simulink model "final"  (R2023a)
settings: Solver=VariableStepAuto  StartTime=0.0  StopTime=1.5  RelTol=1e-3
libraries: dspfdesign x6, spspowerguiLib x1
settings Model: SimulationMode=accelerator  Creator=04  LastModifiedBy=23688
settings SolverCC: AlgebraicLoopSolver=TrustRegion
settings DataIOCC: ReturnWorkspaceOutputs=off
settings DebuggingCC: UnconnectedInputMsg=warning  UnconnectedOutputMsg=warning  UnconnectedLineMsg=warning
settings ModelReferenceCC: EnableRefExpFcnMdlSchedulingChecks=on
settings RTWCC: DLArmComputeVersion=19.05

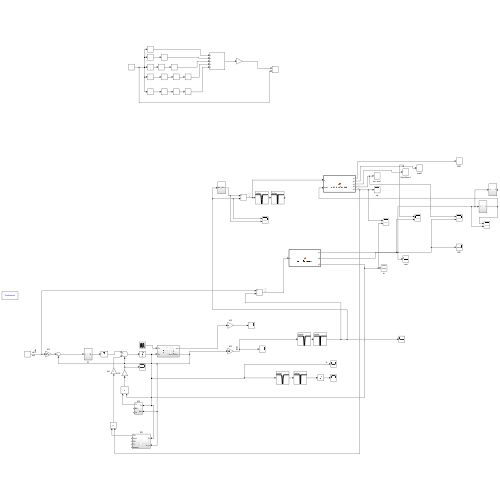
[thumbnail: Simulink's stored preview of the top-level diagram]
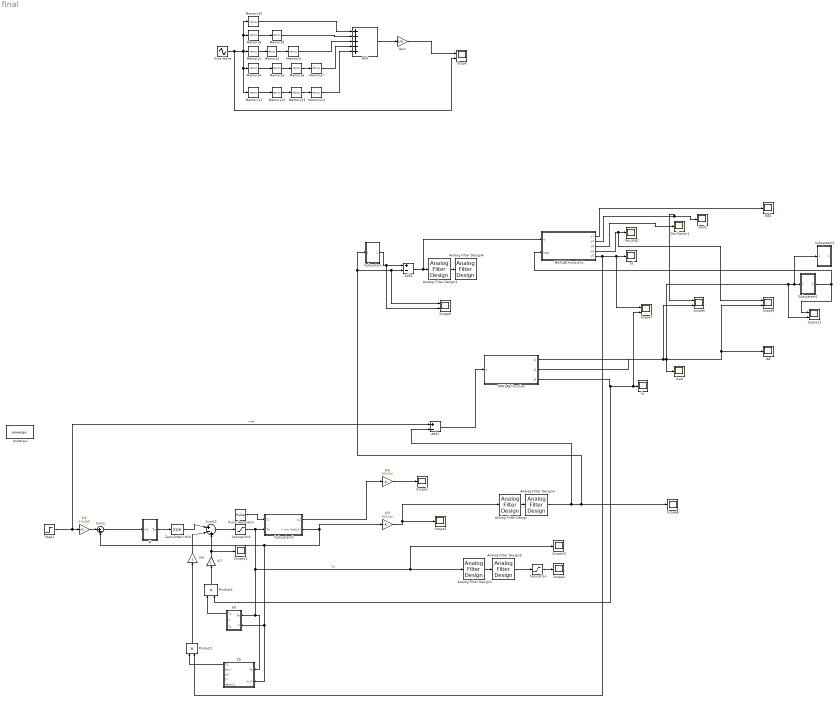
== system final ==
  Add : Sum  Inputs=+++++
  Add1 : Sum  Inputs=+-
  Add2 : Sum  Inputs=+-
  Analog Filter Design : dspfdesign/Analog Filter Design  method=Butterworth  filttype=Bandstop  N=12  Wlo=700*2*pi  Whi=1300*2*pi  Rp=2  Rs=40
  Analog Filter Design1 : dspfdesign/Analog Filter Design  method=Butterworth  filttype=Bandstop  N=2  Wlo=700*2*pi  Whi=1300*2*pi  Rp=2  Rs=40
  Analog Filter Design2 : dspfdesign/Analog Filter Design  method=Butterworth  filttype=Bandstop  N=12  Wlo=700*2*pi  Whi=1300*2*pi  Rp=2  Rs=40
  Analog Filter Design3 : dspfdesign/Analog Filter Design  method=Butterworth  filttype=Bandstop  N=12  Wlo=900*2*pi  Whi=1100*2*pi  Rp=2  Rs=40
  Analog Filter Design4 : dspfdesign/Analog Filter Design  method=Butterworth  filttype=Bandstop  N=12  Wlo=900*2*pi  Whi=1100*2*pi  Rp=2  Rs=40
  Analog Filter Design5 : dspfdesign/Analog Filter Design  method=Butterworth  filttype=Bandstop  N=2  Wlo=950*2*pi  Whi=1050*2*pi  Rp=2  Rs=40
  Gain : Gain  Gain=1/5
  IAE : Scope
  IAE1 : Scope
  Iae_avg1 : Scope
  KR : Subsystem
  Ki2 : Gain  Gain=2*pi/60
  Ki3 : Gain  Gain=60/2/pi
  Ki5 : Gain  Gain=60/2/pi
  Ki6 : Gain
  Ki7 : Gain
  MATLAB Function : MATLAB Function  TreatAsAtomicUnit=on
  MATLAB Function1 : MATLAB Function  TreatAsAtomicUnit=on
  Memory{1..14} (14 alike) : Memory  InitialCondition=0.001
  Oscillation1 : Scope
  PI : Subsystem
  Product1 : Product
  Product2 : Product
  Pulse Generator : DiscretePulseGenerator  PulseType=Time based  Amplitude=2.39*0.5*1  Period=0.8  PulseWidth=50  PhaseDelay=0.4
  Saturation : Saturate  UpperLimit=2.39*3  LowerLimit=-2.39*3  ZeroCross=off
  Saturation3 : Saturate  UpperLimit=2.39*3  LowerLimit=-2.39*3
  Scope{,5..7,9,11} (6 alike) : Scope  NumInputPorts=2
  Scope{1..3,8,10,12} (6 alike) : Scope
  Sine Wave : Sin  Frequency=1000*2*pi  SampleTime=0
  Step2 : Step  Time=0.01  After=1000  SampleTime=0
  Subsystem : Subsystem
  Subsystem1 : Subsystem
  Subsystem2 : Subsystem
  Subsystem3 : Subsystem
  Sum13 : Sum  Inputs=|+-+
  Sum2 : Sum  Inputs=|+-
  ZD : Subsystem
  Zero-Order Hold : ZeroOrderHold  SampleTime=0.0005
  kr : Scope
  load : Scope
  load1 : Scope
  powergui : spspowerguiLib/powergui  Priority=1  SimulationMode=Continuous  SampleTime=50e-6  frequency=60  Iterations=50  frequencyindice=60  Pbase=100e6  ErrMax=1e-4  UnitsV=kV  UnitsW=MW  buscounter=0  FunctionMessages=off  echomessages=off  EnableUseOfTLC=off  CurrentSourceSwitches=off  DisableSnubberDevices=off  DisableRonSwitches=off  DisableVfSwitches=off  DisplayEquations=off  AutomaticDiscreteSolvers=off  SolverType=Tustin/Backward Euler (TBE)  Interpol=off  ExternalGateDelay=off  methode=off  Ts=100  x0status=blocks  SPID=on  SwTol=0  HookPort=off  NonlinearTolerance=1e-4  nMaxIteration=100  ContinueOnMaxIteration=off  RestoreLinks=warning  ResistiveCurrentMeasurement=off  Frange=[0:2:500]  Ylog=off  Xlog=on  ShowGrid=off  save=off  variable=ZData  structure=0  ZoomFFT=off  StartTime=0.0  cycles=1  DisplayStyle=1  fundamental=60  FreqAxis=off  MaxFrequency=1000  frequencyindicesteady=1  RmsSteady=1  display=off
  zd : Scope
  wires:
  Memory1/1 -> Memory2/1
  Memory2/1 -> Memory3/1
  Memory4/1 -> Memory5/1
  Memory5/1 -> Memory6/1
  Memory6/1 -> Memory7/1
  Memory8/1 -> Memory9/1
  Memory10/1 -> Add/1
  Memory9/1 -> Add/2
  Memory3/1 -> Add/3
  Memory7/1 -> Add/4
  Memory14/1 -> Add/5
  Memory13/1 -> Memory14/1
  Memory12/1 -> Memory13/1
  Memory11/1 -> Memory12/1
  Sine Wave/1 -> Scope/2, Memory10/1, Memory8/1, Memory11/1, Memory4/1, Memory1/1
  Add/1 -> Gain/1
  Gain/1 -> Scope/1
  Ki5/1 -> Scope1/1
  Step2/1 -> Add1/1, Ki2/1  "wref"
  Add1/1 -> MATLAB Function/1(e)
  Saturation3/1 -> Subsystem2/2(Te), Scope10/1, Analog Filter Design1/1, ZD/1(Te), KR/1(Te)  "Te"
  MATLAB Function/1(y1) -> IAE/1, Scope6/2
  Analog Filter Design/1 -> Analog Filter Design3/1
  Sum13/1 -> Saturation3/1
  Ki7/1 -> Sum13/3, Scope12/1
  Product1/1 -> Ki6/1
  Ki6/1 -> Sum13/2
  Product2/1 -> Ki7/1
  Ki3/1 -> Analog Filter Design/1, Scope3/1
  Ki2/1 -> Sum2/1
  MATLAB Function1/2(y2) -> Scope5/1, load1/1
  MATLAB Function1/3(y3) -> Oscillation1/1
  MATLAB Function1/4(y4) -> Scope6/1, Iae_avg1/1
  MATLAB Function1/1(y1) -> IAE1/1
  MATLAB Function1/5(y5) -> Scope7/1, zd/1, Product1/2
  Analog Filter Design2/1 -> Analog Filter Design4/1
  Add2/1 -> MATLAB Function1/1(e), Analog Filter Design2/1
  MATLAB Function/3(y3) -> Scope7/2, kr/1, Product2/2
  Subsystem/1(wm_filter) -> Scope9/2, Add2/1
  Analog Filter Design3/1 -> Scope8/1, Scope9/1, Add2/2, Subsystem/1(In1), Add1/2
  MATLAB Function/2(y2) -> Scope5/2, load/1, Scope11/2, Subsystem3/1(In1), Subsystem1/1(In1)
  Subsystem1/1(Out1) -> Scope11/1, MATLAB Function1/2(load)
  Analog Filter Design1/1 -> Analog Filter Design5/1
  Analog Filter Design5/1 -> Saturation/1
  Saturation/1 -> Scope2/1
  Sum2/1 -> PI/1(In1)
  Subsystem2/2(< wm (rad/s)>) -> Ki3/1, Sum2/2, ZD/2(w_m), KR/2(Wm)
  Pulse Generator/1 -> Subsystem2/1(TL)
  Subsystem2/1(w2) -> Ki5/1
  KR/1(TL) -> Product2/1
  ZD/1(TS) -> Product1/1
  PI/1(Te) -> Zero-Order Hold/1
  Zero-Order Hold/1 -> Sum13/1

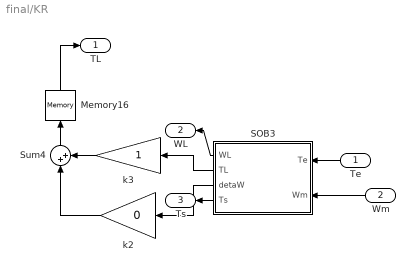
== system final/KR ==
  Te : Inport
  Wm : Inport  Port=2
  Memory16 : Memory
  SOB3 : Subsystem
  Sum4 : Sum  Inputs=|++
  k2 : Gain  Gain=0
  k3 : Gain
  TL : Outport
  WL : Outport  Port=2
  Ts : Outport  Port=3
  wires:
  Sum4/1 -> Memory16/1
  Memory16/1 -> TL/1
  SOB3/3(detaW) -> k2/1
  SOB3/1(WL) -> WL/1
  SOB3/4(Ts) -> Ts/1
  SOB3/2(TL) -> k3/1
  k3/1 -> Sum4/2
  k2/1 -> Sum4/1
  Wm/1 -> SOB3/2(Wm)
  Te/1 -> SOB3/1(Te)

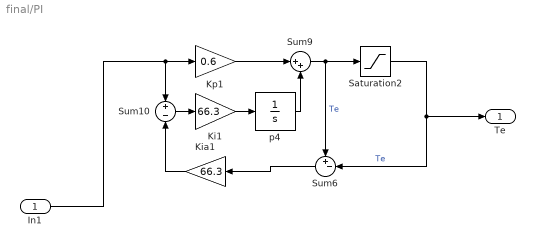
== system final/PI ==
  In1 : Inport
  Ki1 : Gain  Gain=66.3
  Kia1 : Gain  Gain=66.3
  Kp1 : Gain  Gain=0.6
  Saturation2 : Saturate  UpperLimit=2.39*3  LowerLimit=-2.39*3
  Sum10 : Sum  Inputs=+|-
  Sum6 : Sum  Inputs=+-|
  Sum9 : Sum  Inputs=|++
  p4 : TransferFcn  Denominator=[1 0]
  Te : Outport
  wires:
  Kia1/1 -> Sum10/2
  Sum6/1 -> Kia1/1
  Sum10/1 -> Ki1/1
  Kp1/1 -> Sum9/1
  Saturation2/1 -> Te/1, Sum6/2  "Te"
  Sum9/1 -> Sum6/1, Saturation2/1  "Te"
  p4/1 -> Sum9/2
  Ki1/1 -> p4/1
  In1/1 -> Kp1/1, Sum10/1

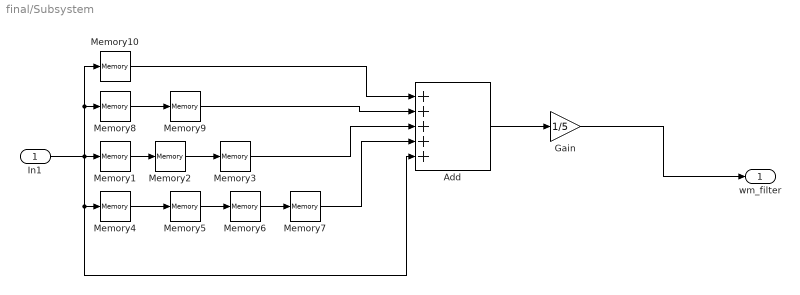
== system final/Subsystem ==
  In1 : Inport
  Add : Sum  Inputs=+++++
  Gain : Gain  Gain=1/5
  Memory{1..10} (10 alike) : Memory
  wm_filter : Outport
  wires:
  In1/1 -> Memory10/1, Memory8/1, Add/5, Memory4/1, Memory1/1
  Memory1/1 -> Memory2/1
  Memory4/1 -> Memory5/1
  Add/1 -> Gain/1
  Memory8/1 -> Memory9/1
  Memory5/1 -> Memory6/1
  Memory9/1 -> Add/2
  Memory7/1 -> Add/4
  Memory6/1 -> Memory7/1
  Memory10/1 -> Add/1
  Memory3/1 -> Add/3
  Memory2/1 -> Memory3/1
  Gain/1 -> wm_filter/1

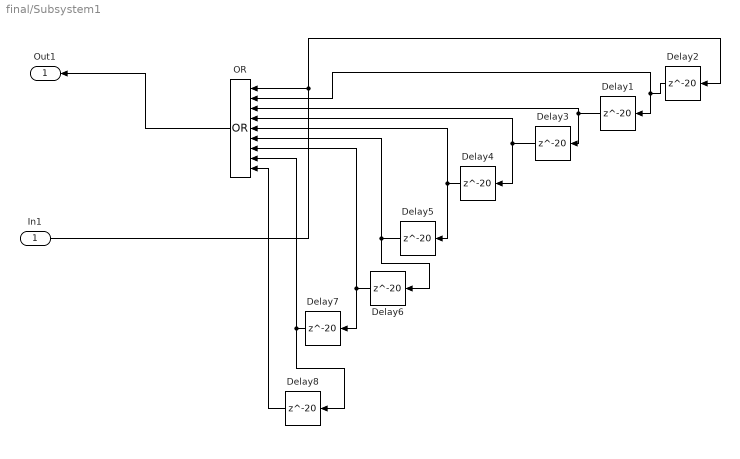
== system final/Subsystem1 ==
  In1 : Inport
  Delay{1..8} (8 alike) : Delay  DelayLength=20
  OR : Logic  Operator=OR  Inputs=9  IconShape=distinctive  AllPortsSameDT=off  OutDataTypeStr=boolean
  Out1 : Outport
  wires:
  Delay2/1 -> Delay1/1, OR/2
  Delay4/1 -> Delay5/1, OR/5
  Delay3/1 -> Delay4/1, OR/4
  Delay1/1 -> OR/3, Delay3/1
  In1/1 -> Delay2/1, OR/1
  OR/1 -> Out1/1
  Delay5/1 -> Delay6/1, OR/6
  Delay6/1 -> Delay7/1, OR/7
  Delay7/1 -> Delay8/1, OR/8
  Delay8/1 -> OR/9

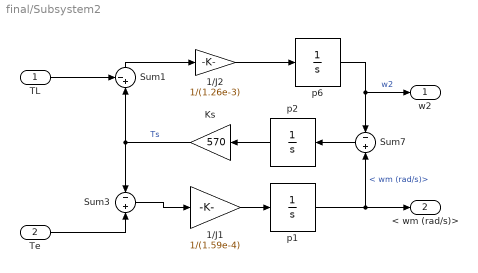
== system final/Subsystem2 ==
  TL : Inport
  Te : Inport  Port=2
  1/J1 : Gain  Gain=1/(1.59e-4)
  1/J2 : Gain  Gain=1/(1.26e-3)
  Ks : Gain  Gain=570
  Sum1 : Sum  Inputs=-+|
  Sum3 : Sum  Inputs=-+
  Sum7 : Sum  Inputs=-+
  p1 : TransferFcn  Denominator=[1 0]
  p2 : TransferFcn  Denominator=[1 0]
  p6 : TransferFcn  Denominator=[1 0]
  w2 : Outport
  < wm (rad/s)> : Outport  Port=2
  wires:
  Sum3/1 -> 1/J1/1
  1/J1/1 -> p1/1
  p1/1 -> < wm (rad/s)>/1, Sum7/2  "< wm (rad/s)>"
  p6/1 -> w2/1, Sum7/1  "w2"
  Sum7/1 -> p2/1
  Sum1/1 -> 1/J2/1
  Ks/1 -> Sum3/1, Sum1/2  "Ts"
  p2/1 -> Ks/1
  1/J2/1 -> p6/1
  TL/1 -> Sum1/1
  Te/1 -> Sum3/2

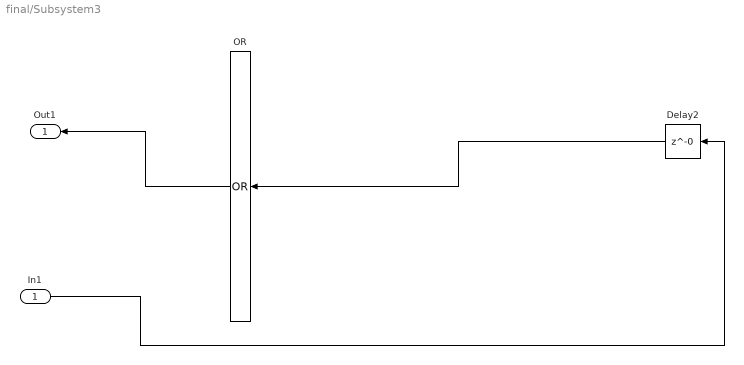
== system final/Subsystem3 ==
  In1 : Inport
  Delay2 : Delay  DelayLength=0
  OR : Logic  Operator=OR  Inputs=1  IconShape=distinctive  AllPortsSameDT=off  OutDataTypeStr=boolean
  Out1 : Outport
  wires:
  OR/1 -> Out1/1
  Delay2/1 -> OR/1
  In1/1 -> Delay2/1

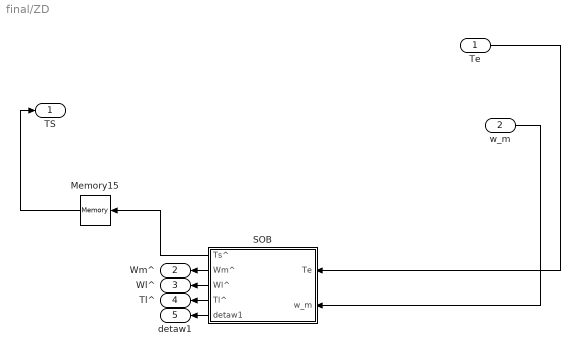
== system final/ZD ==
  Te : Inport
  w_m : Inport  Port=2
  Memory15 : Memory
  SOB : Subsystem
  TS : Outport
  Wm^ : Outport  Port=2
  Wl^ : Outport  Port=3
  Tl^ : Outport  Port=4
  detaw1 : Outport  Port=5
  wires:
  SOB/4(Tl^) -> Tl^/1
  SOB/1(Ts^) -> Memory15/1
  Memory15/1 -> TS/1
  w_m/1 -> SOB/2(w_m)
  SOB/2(Wm^) -> Wm^/1
  Te/1 -> SOB/1(Te)
  SOB/5(detaw1) -> detaw1/1
  SOB/3(Wl^) -> Wl^/1

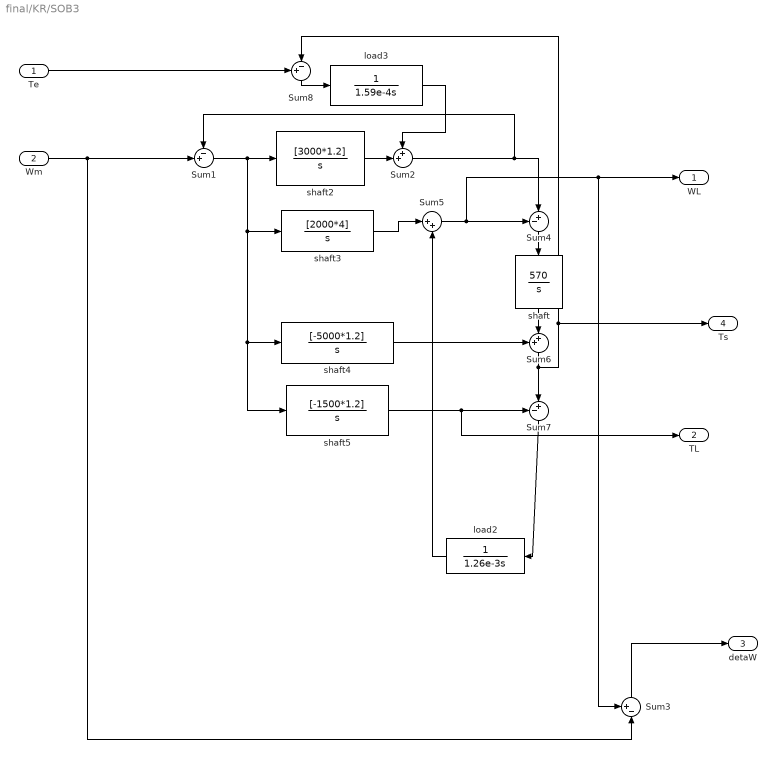
== system final/KR/SOB3 ==
  Te : Inport
  Wm : Inport  Port=2
  Sum1 : Sum  Inputs=-+|
  Sum2 : Sum  Inputs=++|
  Sum3 : Sum  Inputs=+-|
  Sum4 : Sum  Inputs=-+|
  Sum5 : Sum  Inputs=|++
  Sum6 : Sum  Inputs=++|
  Sum7 : Sum  Inputs=-+|
  Sum8 : Sum  Inputs=+-|
  load2 : TransferFcn  Denominator=[1.26e-3 0]
  load3 : TransferFcn  Denominator=[1.59e-4 0]
  shaft : TransferFcn  Numerator=[570]  Denominator=[1 0]
  shaft2 : TransferFcn  Numerator=[3000*1.2]  Denominator=[1 0]
  shaft3 : TransferFcn  Numerator=[2000*4]  Denominator=[1 0]
  shaft4 : TransferFcn  Numerator=[-5000*1.2]  Denominator=[1 0]
  shaft5 : TransferFcn  Numerator=[-1500*1.2]  Denominator=[1 0]
  WL : Outport  VectorParamsAs1DForOutWhenUnconnected=off
  TL : Outport  Port=2  VectorParamsAs1DForOutWhenUnconnected=off
  detaW : Outport  Port=3  VectorParamsAs1DForOutWhenUnconnected=off
  Ts : Outport  Port=4  VectorParamsAs1DForOutWhenUnconnected=off
  wires:
  Wm/1 -> Sum1/2, Sum3/2
  Te/1 -> Sum8/1
  load3/1 -> Sum2/1
  Sum8/1 -> load3/1
  load2/1 -> Sum5/2
  Sum7/1 -> load2/1
  Sum6/1 -> Sum7/2, Ts/1, Sum8/2
  shaft5/1 -> TL/1, Sum7/1
  shaft/1 -> Sum6/2
  shaft4/1 -> Sum6/1
  Sum4/1 -> shaft/1
  Sum5/1 -> WL/1, Sum3/1, Sum4/1
  shaft3/1 -> Sum5/1
  Sum2/1 -> Sum4/2, Sum1/1
  shaft2/1 -> Sum2/2
  Sum1/1 -> shaft5/1, shaft4/1, shaft3/1, shaft2/1
  Sum3/1 -> detaW/1

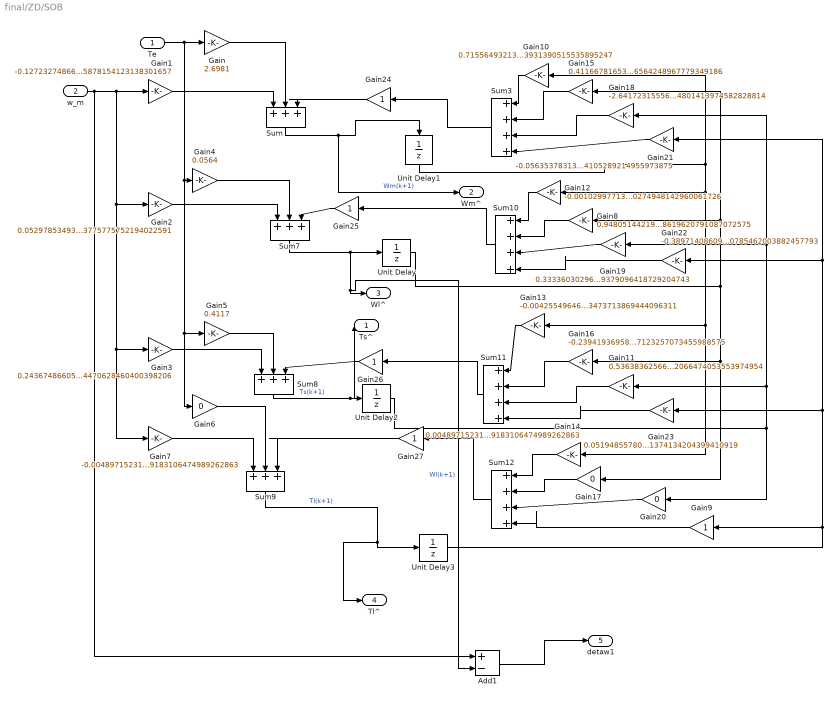
== system final/ZD/SOB ==
  Te : Inport
  w_m : Inport  Port=2
  Add1 : Sum  Inputs=+-
  Gain : Gain  Gain=2.6981
  Gain1 : Gain  Gain=-0.12723274866755878154123138301657
  Gain10 : Gain  Gain=0.7155649321343931390515535895247
  Gain11 : Gain  Gain=0.53638362566622066474053553974954
  Gain12 : Gain  Gain=-0.0010299771306700274948142960061726
  Gain13 : Gain  Gain=-0.004255496467973473713869444096311
  Gain14 : Gain  Gain=0.0048971523131869183106474989262863
  Gain15 : Gain  Gain=0.41166781653316564248967779349186
  Gain16 : Gain  Gain=-0.23941936958917123257073455988575
  Gain17 : Gain  Gain=0
  Gain18 : Gain  Gain=-2.6417231555684801413974582828814
  Gain19 : Gain  Gain=0.33336030296459379096418729204743
  Gain2 : Gain  Gain=0.052978534931283775775752194022591
  Gain20 : Gain  Gain=0
  Gain21 : Gain  Gain=-0.056353783132214105289214955973875
  Gain22 : Gain  Gain=-0.38971408609680785462003882457793
  Gain23 : Gain  Gain=0.05194855780061374134204399410919
  Gain{9,24..27} (5 alike) : Gain
  Gain3 : Gain  Gain=0.24367486605714470628460400398206
  Gain4 : Gain  Gain=0.0564
  Gain5 : Gain  Gain=0.4117
  Gain6 : Gain  Gain=0
  Gain7 : Gain  Gain=-0.0048971523131869183106474989262863
  Gain8 : Gain  Gain=0.94805144219938619620791087072575
  Sum{,7..9} (4 alike) : Sum  Inputs=+++|
  Sum{3,10..12} (4 alike) : Sum  Inputs=++++|
  Unit Delay{,1..3} (4 alike) : UnitDelay  SampleTime=-1
  Ts^ : Outport
  Wm^ : Outport  Port=2
  Wl^ : Outport  Port=3
  Tl^ : Outport  Port=4
  detaw1 : Outport  Port=5
  wires:
  Te/1 -> Gain5/1, Gain6/1, Gain4/1, Gain/1
  Gain/1 -> Sum/2
  Gain1/1 -> Sum/1
  Gain4/1 -> Sum7/2
  Gain2/1 -> Sum7/1
  Gain5/1 -> Sum8/2
  Gain3/1 -> Sum8/1
  Gain6/1 -> Sum9/2
  Gain7/1 -> Sum9/1
  Sum/1 -> Unit Delay1/1, Wm^/1  "Wm(k+1)"
  Sum7/1 -> Add1/2, Wl^/1, Unit Delay/1  "Wl(k+1)"
  Sum8/1 -> Ts^/1, Unit Delay2/1  "Ts(k+1)"
  Sum9/1 -> Tl^/1, Unit Delay3/1  "Tl(k+1)"
  Sum12/1 -> Gain27/1
  Gain10/1 -> Sum3/1
  Gain11/1 -> Sum11/3
  Gain9/1 -> Sum12/4
  Gain12/1 -> Sum10/1
  Gain13/1 -> Sum11/1
  Gain14/1 -> Sum12/1
  Gain17/1 -> Sum12/2
  Gain19/1 -> Sum10/3
  Unit Delay1/1 -> Gain14/1, Gain13/1, Gain12/1, Gain10/1
  Unit Delay/1 -> Gain8/1, Gain15/1, Gain17/1, Gain16/1
  Unit Delay2/1 -> Gain11/1, Gain18/1, Gain19/1, Gain20/1
  Unit Delay3/1 -> Gain21/1, Gain22/1, Gain23/1, Gain9/1
  Gain25/1 -> Sum7/3
  Gain26/1 -> Sum8/3
  Sum3/1 -> Gain24/1
  Gain24/1 -> Sum/3
  Gain15/1 -> Sum3/2
  Gain18/1 -> Sum3/3
  Gain21/1 -> Sum3/4
  Sum10/1 -> Gain25/1
  Gain8/1 -> Sum10/2
  Sum11/1 -> Gain26/1
  Gain16/1 -> Sum11/2
  Gain23/1 -> Sum11/4
  Gain27/1 -> Sum9/3
  Gain20/1 -> Sum12/3
  Gain22/1 -> Sum10/4
  Add1/1 -> detaw1/1
  w_m/1 -> Add1/1, Gain3/1, Gain7/1, Gain2/1, Gain1/1

== matlab function final/MATLAB Function ==
  settings: updateMethod=DISCRETE
  data: y1 output; y2 output; e input; y3 output
function [y1,y2,y3]= anti_interference(e)
persistent zd kr IAE IAE_lim  h e_old load t IAE_lim_so IAE_sum num IAE_average oscillation
%initialization
if isempty(num)
 num=0;      %幅值
end
%if isempty(Ti)
 %Ti=0.25;  %积分时间常数
%end
if isempty(h)
 h=0.0005;    %采样周期
end
if isempty(IAE)
 IAE=0;    %面积
end
if isempty(IAE_average)
    IAE_average=0;
end
if isempty(load)
 load=0;   %用于判断否存在干扰
end
if isempty(e_old)
 e_old=0;  %上一采样时刻误差
end
if isempty(t)
    t=0;
end

if isempty(IAE_lim)
    IAE_lim=0.08;
  % IAE_lim=2*a/Ti;   %用于判断振荡的临界值
end

if isempty(oscillation)
    oscillation=0;  %面积最大值
end
if isempty(IAE_sum)
    IAE_sum=0;  %面积最大值
end
if isempty(zd)
    zd=0;  %面积最大值
end
if isempty(kr)
    kr=0;  %面积最大值
end

% LOAD DETECTION 
if (t>=0.6)
  if sign(e)==sign(e_old)
     IAE=IAE+abs(e)*h;
     if IAE>IAE_lim
         load=1;
     else
         load =0;
     end
  else
        load=0;
      IAE=0;
  end
  
else
    t=t+h;  
end
   e_old=e;


if(load==1)
    
        kr=kr+0.01; 
        
end     
if(load==0)
%    
%     if(kr>=0.001)
%         kr=kr-0.001;
%     end
%     if(kr<=-0.001)
%         kr=kr+0.001;
%        
%     end
end
y1=IAE;
y2=load;
y3=kr;

== matlab function final/MATLAB Function1 ==
  settings: updateMethod=DISCRETE
  data: y1 output; y2 output; e input; y3 output; y4 output; y5 output; load input
function [y1,y2,y3,y4,y5]= anti_interference(e,load)
persistent zd kr IAE  h e_old  t IAE_lim_so IAE_sum num IAE_average oscillation
%initialization
if isempty(num)
 num=0;      %幅值
end
%if isempty(Ti)
 %Ti=0.25;  %积分时间常数
%end
if isempty(h)
 h=0.0005;    %采样周期
end
if isempty(IAE)
 IAE=0;    %面积
end
if isempty(IAE_average)
    IAE_average=0;
end

if isempty(e_old)
 e_old=0;  %上一采样时刻误差
end
if isempty(t)
    t=0;
end

if isempty(IAE_lim_so)
    IAE_lim_so=0.00015;
  % IAE_lim=2*a/Ti;   %用于判断振荡的临界值
end
if isempty(oscillation)
    oscillation=0;  %面积最大值
end
if isempty(IAE_sum)
    IAE_sum=0;  %面积最大值
end
if isempty(zd)
    zd=0;  %面积最大值
end
if isempty(kr)
    kr=0;  %面积最大值
end

% LOAD DETECTION 
if (t>=0.5)
  if sign(e)==sign(e_old)
     IAE=IAE+abs(e)*h;
    
  else
        num=num+1;
       IAE_sum=IAE_sum+IAE;%总面积
        IAE=0;
  end
    %OSCILLATION DETECTION 
    if num==4
        IAE_average=IAE_sum/3;
          IAE_sum=0;
           num=0;

    else
        IAE_average=0;

    end
    if IAE_average>IAE_lim_so
           oscillation=1;
       else
           oscillation=0;
    end  
  
else
    t=t+h;  
end
   e_old=e;
  %OSCILLATION-LOAD
if (oscillation==1&&load==0)
    
    zd=zd+0.2;
end
if(load==1)
%          IAE_average=0;
%          IAE_sum=0;
%          num=0;

end     
y1=IAE;
y2=load;
y3=oscillation;
y4=IAE_average;
y5=zd;
